simulink model "pll_1"  (Simulink 4.00)
settings: Solver=ode45  SolverMode=SingleTasking  StartTime=0.0  StopTime=10.0  RelTol=1e-3  AbsTol=1e-6
values from neighbouring files (symbols this model uses):
  f0 = 500    [chirp_1.m]    (also in costas1f.m = pf0; op_freq.m = 15; pll_5f.m = f01)
  kvco = pkvco    [costas1f.m]    (also in pll_5f.m = kvco1)
  tau = ptau    [costas1f.m]    (also in op_freq.m = 0.0106103295395; pll_5f.m = tau1)
settings Model: LastModifiedBy=Administrator  LimitDataPoints=off  BlockReductionOpt=off

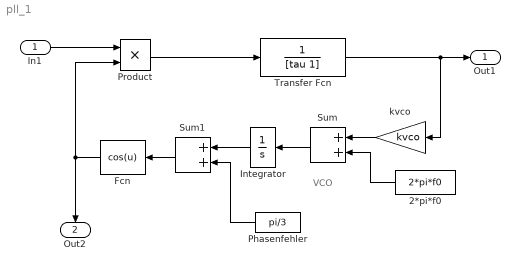
== system pll_1 ==
  note: VCO
  In1 : Inport  Port=1
  2*pi*f0 : Constant  Orientation=left  Value=2*pi*f0
  Fcn : Fcn  Orientation=left  Expr=cos(u)
  Integrator : Integrator  Orientation=left  ExternalReset=none  InitialConditionSource=internal  InitialCondition=0  LimitOutput=off  UpperSaturationLimit=inf  LowerSaturationLimit=-inf  ShowSaturationPort=off  ShowStatePort=off  AbsoluteTolerance=auto
  Phasenfehler : Constant  Orientation=left  Value=pi/3
  Product : Product  Inputs=2  Multiplication=Element-wise(.*)  SaturateOnIntegerOverflow=on
  Sum : Sum  Orientation=left  Inputs=++  SaturateOnIntegerOverflow=on
  Sum1 : Sum  Orientation=left  Inputs=++  SaturateOnIntegerOverflow=on
  Transfer Fcn : TransferFcn  Numerator=[1]  Denominator=[tau 1]  Realization=auto  AbsoluteTolerance=auto
  kvco : Gain  Orientation=left  Gain=kvco  Multiplication=Element-wise(K.*u)  SaturateOnIntegerOverflow=on
  Out1 : Outport  Port=1
  Out2 : Outport  Orientation=down  Port=2
  wires:
  In1/1 -> Product/1
  Product/1 -> Transfer Fcn/1
  Transfer Fcn/1 -> kvco/1, Out1/1
  Fcn/1 -> Product/2, Out2/1
  Sum/1 -> Integrator/1
  2*pi*f0/1 -> Sum/2
  kvco/1 -> Sum/1
  Sum1/1 -> Fcn/1
  Integrator/1 -> Sum1/1
  Phasenfehler/1 -> Sum1/2
